simulink model "ej1"  (R2023a)
settings: Solver=VariableStepAuto  StartTime=0.0  StopTime=70  MaxStep=1e-4  RelTol=1e-3
libraries: SignalEditorBlockLib x2
settings Model: Creator=Juan  LastModifiedBy=Juan

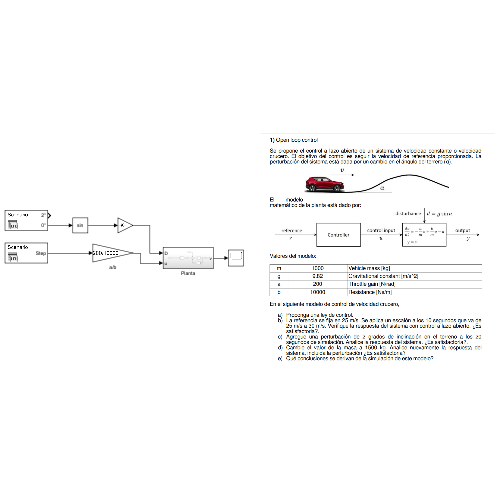
[thumbnail: Simulink's stored preview of the top-level diagram]
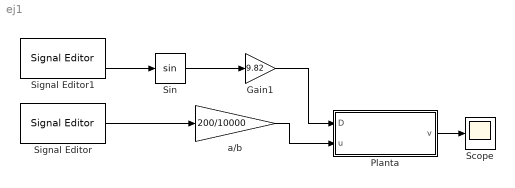
== system ej1 ==
  Gain1 : Gain  Gain=9.82
  Planta : Subsystem
  Scope : Scope
  Signal Editor : SignalEditorBlockLib/Signal Editor  FileName=D:\01. Facultad\Control y Sistemas1\Control y Sistemas\Tp8\v_ref.mat  ActiveScenario=Scenario  ActiveSignal=Step  IsBus=off  OutputBusObjectStr=Bus: BusObject  SampleTime=0  Interpolate=off  ZeroCross=off  OutputAfterFinalValue=Setting to zero  Unit=inherit  PreserveSignalName=on  ApplySigPropsToAllScenarios=on
  Signal Editor1 : SignalEditorBlockLib/Signal Editor  FileName=D:\01. Facultad\Control y Sistemas1\Control y Sistemas\Tp8\perturbn.mat  ActiveScenario=Scenario  ActiveSignal=2°  IsBus=off  OutputBusObjectStr=Bus: BusObject  SampleTime=0  Interpolate=off  ZeroCross=off  OutputAfterFinalValue=Setting to zero  Unit=inherit  PreserveSignalName=on  ApplySigPropsToAllScenarios=on
  Sin : Trigonometry
  a/b : Gain  Gain=200/10000
  wires:
  Signal Editor/1 -> a/b/1
  Signal Editor1/2 -> Sin/1
  Planta/1(v) -> Scope/1
  Sin/1 -> Gain1/1
  Gain1/1 -> Planta/1(D)
  a/b/1 -> Planta/2(u)

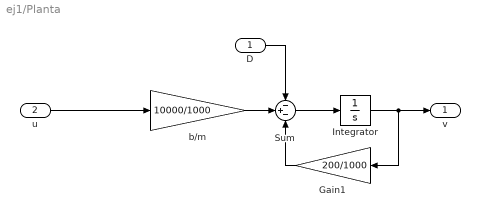
== system ej1/Planta ==
  D : Inport
  u : Inport  Port=2
  Gain1 : Gain  Gain=200/1000
  Integrator : Integrator  InitialCondition=25
  Sum : Sum  Inputs=-+-
  b/m : Gain  Gain=10000/1000
  v : Outport
  wires:
  u/1 -> b/m/1
  b/m/1 -> Sum/2
  D/1 -> Sum/1
  Sum/1 -> Integrator/1
  Gain1/1 -> Sum/3
  Integrator/1 -> Gain1/1, v/1
